simulink subsystem "MotorsDCFaulhaber_2342S_012_CR"  (R2023b)
settings: Solver=VariableStepAuto  StartTime=0.0  StopTime=10.0  RelTol=1e-3
undefined symbols (not defined in the file): Motor1, Motor2, Motor3, Phase1_Pos, Phase2_Pos, Phase3_Pos, Phase_Neg, Reference
libraries: fl_lib x1
settings Model: DataDictionary=neck_mk3.sldd  EnableAccessToBaseWorkspace=off  Creator=upattacini  LastModifiedBy=upattacini

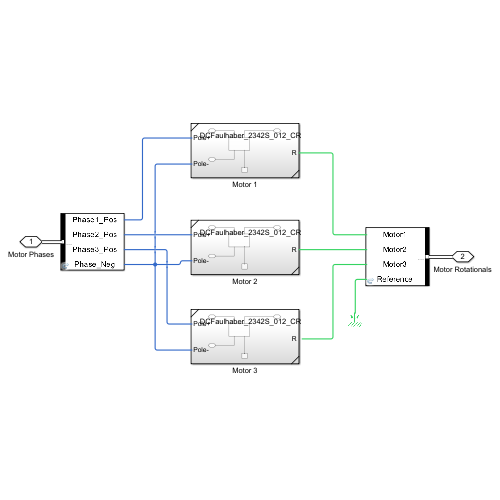
[thumbnail: Simulink's stored preview of the top-level diagram]
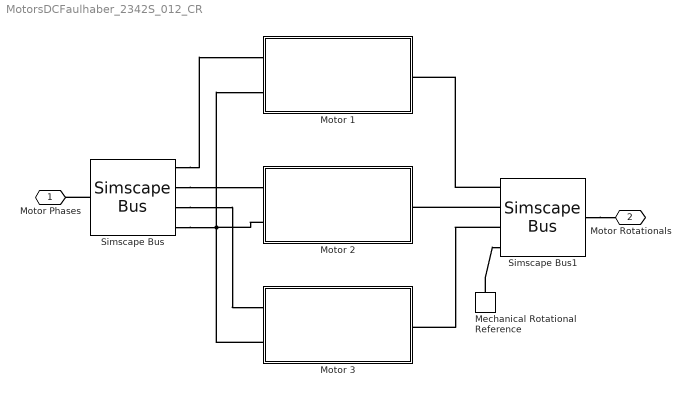
== system MotorsDCFaulhaber_2342S_012_CR ==
  Mechanical Rotational Reference : fl_lib/Mechanical/Rotational Elements/Mechanical Rotational Reference
  Motor 1 : Subsystem  ReferencedSubsystem=DCFaulhaber_2342S_012_CR
      settings: PermitHierarchicalResolution=None
  Motor 2 : Subsystem  ReferencedSubsystem=DCFaulhaber_2342S_012_CR
      settings: PermitHierarchicalResolution=None
  Motor 3 : Subsystem  ReferencedSubsystem=DCFaulhaber_2342S_012_CR
      settings: PermitHierarchicalResolution=None
  Simscape Bus : SimscapeBus  HierarchyStrings=Phase1_Pos;Phase2_Pos;Phase3_Pos;Phase_Neg  ConnectionType=Bus: Physical_MotorPhases
  Simscape Bus1 : SimscapeBus  HierarchyStrings=Motor1;Motor2;Motor3;Reference  ConnectionType=Bus: Physical_MotorRotationals
  Motor Phases : PMIOPort  Side=Left
  Motor Rotationals : PMIOPort  Port=2  Side=Right
  connections:
  Motor 2/LConn2 -- Motor 3/LConn2 -- Simscape Bus/LConn4 -- Motor 1/LConn2
  Simscape Bus/RConn1 -- Motor Phases/RConn1
  Simscape Bus1/RConn1 -- Motor Rotationals/RConn1
  Simscape Bus1/LConn1 -- Motor 1/RConn1
  Simscape Bus1/LConn3 -- Motor 3/RConn1
  Simscape Bus1/LConn2 -- Motor 2/RConn1
  Simscape Bus/LConn1 -- Motor 1/LConn1
  Simscape Bus/LConn2 -- Motor 2/LConn1
  Simscape Bus/LConn3 -- Motor 3/LConn1
  Mechanical Rotational Reference/LConn1 -- Simscape Bus1/LConn4
